simulink model "sim2"  (R2021a)
settings: Solver=ode4  StartTime=0.0  StopTime=2  RelTol=1e-3
libraries: spsVoltageMeasurementLib x7, spsIGBTDiodeLib x6, spsSeriesRLCBranchLib x5, spsCurrentMeasurementLib x4, spsACVoltageSourceLib x3, spsabctodq0Lib x2, spsGroundLib x2, simulink x1, spsdq0toabcLib x1, spspowerguiLib x1
settings Model: Creator=aks  LastModifiedBy=aks
settings SolverCC: ZeroCrossControl=DisableAll
settings DataIOCC: Refine=100

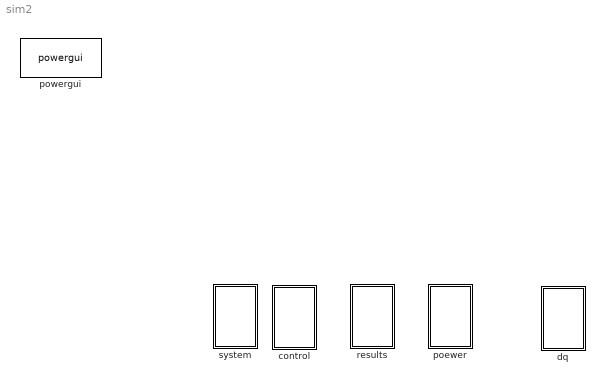
== system sim2 ==
  control : Subsystem
  dq : Subsystem
  poewer : Subsystem
  powergui : spspowerguiLib/powergui  Priority=1  SimulationMode=Discrete  SampleTime=1e-6  frequency=60  Iterations=50  frequencyindice=50  Pbase=100e6  ErrMax=1e-4  UnitsV=kV  UnitsW=MW  buscounter=0  FunctionMessages=off  echomessages=off  EnableUseOfTLC=off  CurrentSourceSwitches=off  DisableSnubberDevices=off  DisableRonSwitches=off  DisableVfSwitches=off  DisplayEquations=off  AutomaticDiscreteSolvers=off  SolverType=Tustin/Backward Euler (TBE)  Interpol=off  ExternalGateDelay=off  methode=off  Ts=100  x0status=blocks  SPID=on  SwTol=0  HookPort=off  NonlinearTolerance=1e-4  nMaxIteration=100  ContinueOnMaxIteration=off  RestoreLinks=warning  ResistiveCurrentMeasurement=off  Frange=[0:2:500]  Ylog=off  Xlog=on  ShowGrid=off  save=off  variable=ZData  structure=0  ZoomFFT=off  StartTime=0.0  cycles=1  DisplayStyle=1  fundamental=60  FreqAxis=off  MaxFrequency=1000  frequencyindicesteady=1  RmsSteady=1  display=off
  results : Subsystem
  system : Subsystem

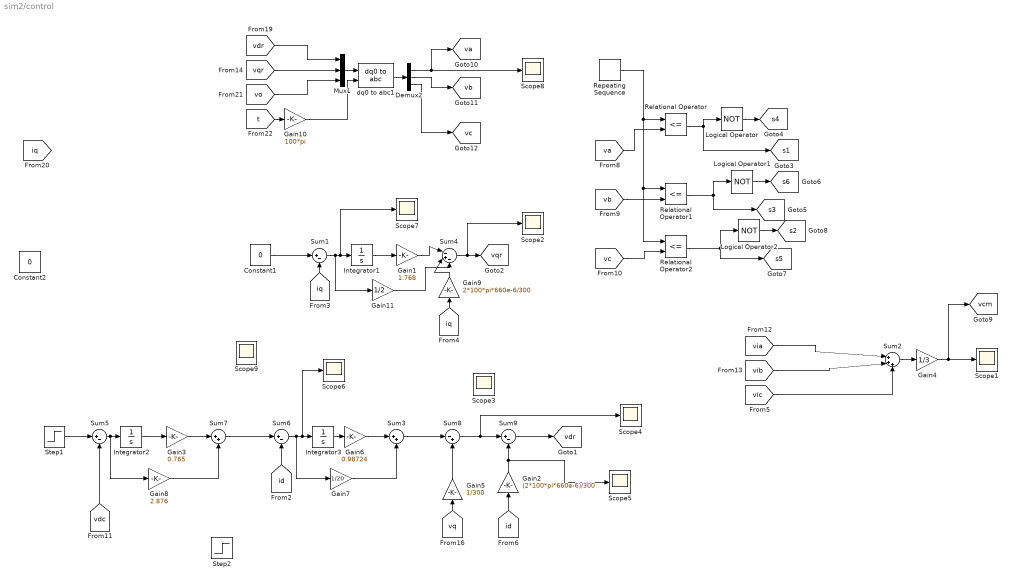
== system sim2/control ==
  Constant1 : Constant  Value=0
  Constant2 : Constant  Value=0
  Demux2 : Demux  Outputs=3
  Gain1 : Gain  Gain=1.768
  Gain10 : Gain  Gain=100*pi
  Gain11 : Gain  Gain=1/2
  Gain2 : Gain  Gain=(2*100*pi*660e-6)/300
  Gain3 : Gain  Gain=0.765
  Gain4 : Gain  Gain=1/3
  Gain5 : Gain  Gain=1/300
  Gain6 : Gain  Gain=0.98724
  Gain7 : Gain  Gain=1/20
  Gain8 : Gain  Gain=2.876
  Gain9 : Gain  Gain=2*100*pi*660e-6/300
  Integrator1 : Integrator
  Integrator2 : Integrator
  Integrator3 : Integrator
  Logical Operator : Logic  Operator=NOT  AllPortsSameDT=off  OutDataTypeStr=boolean
  Logical Operator1 : Logic  Operator=NOT  AllPortsSameDT=off  OutDataTypeStr=boolean
  Logical Operator2 : Logic  Operator=NOT  AllPortsSameDT=off  OutDataTypeStr=boolean
  Mux1 : Mux  Inputs=3
  Relational Operator : RelationalOperator  Operator=<=  OutDataTypeStr=boolean  RndMeth=Simplest
  Relational Operator1 : RelationalOperator  Operator=<=  OutDataTypeStr=boolean  RndMeth=Simplest
  Relational Operator2 : RelationalOperator  Operator=<=  OutDataTypeStr=boolean  RndMeth=Simplest
  Repeating Sequence : simulink/Sources/Repeating Sequence  rep_seq_t=[0 (1/20000) (1/10000) (3/20000) (1/5000)]  rep_seq_y=[0 1 0 -1 0]
  Scope{1..9} (9 alike) : Scope
  Step1 : Step  Before=800  After=400  SampleTime=0
  Step2 : Step  Before=0.4  After=0.6  SampleTime=0
  Sum{1,5..6,9} (4 alike) : Sum  Inputs=|+-
  Sum2 : Sum  Inputs=|+++
  Sum3 : Sum  Inputs=|++
  Sum4 : Sum  Inputs=|-+-
  Sum7 : Sum  Inputs=|++
  Sum8 : Sum  Inputs=|-+
  dq0 to abc1 : spsdq0toabcLib/dq0 to abc  Alignment=90 degrees behind phase A axis
  tag scope: s1=global, s2=global, s3=global, s4=global, s5=global, s6=global, va=global, vb=global, vc=global, vcm=global, vdr=global, vqr=global
  wires:
  Sum1/1 -> Gain11/1, Scope7/1, Integrator1/1
  Integrator1/1 -> Gain1/1
  Gain1/1 -> Sum4/1
  Constant1/1 -> Sum1/1
  Repeating Sequence/1 -> Relational Operator2/1, Relational Operator1/1, Relational Operator/1
  Relational Operator/1 -> [s1], Logical Operator/1
  Logical Operator/1 -> [s4]
  Logical Operator1/1 -> [s6]
  Relational Operator1/1 -> Logical Operator1/1, [s3]
  Relational Operator2/1 -> Logical Operator2/1, [s5]
  Logical Operator2/1 -> [s2]
  Step1/1 -> Sum5/1
  [vdc] -> Sum5/2
  [id] -> Gain2/1
  [iq] -> Gain9/1
  Gain9/1 -> Sum4/2
  Sum6/1 -> Gain7/1, Scope6/1, Integrator3/1
  Integrator3/1 -> Gain6/1
  Sum8/1 -> Scope4/1, Sum9/1
  Gain2/1 -> Scope5/1, Sum9/2
  Gain5/1 -> Sum8/2
  Sum5/1 -> Gain8/1, Integrator2/1
  Integrator2/1 -> Gain3/1
  [vic] -> Sum2/3
  [vib] -> Sum2/2
  [via] -> Sum2/1
  Sum2/1 -> Gain4/1
  Gain4/1 -> [vcm], Scope1/1
  [t] -> Gain10/1
  dq0 to abc1/1 -> Demux2/1
  Gain10/1 -> dq0 to abc1/2
  [vo] -> Mux1/3
  Mux1/1 -> dq0 to abc1/1
  Demux2/1 -> Scope8/1, [va]
  Demux2/2 -> [vb]
  Demux2/3 -> [vc]
  [va] -> Relational Operator/2
  [vb] -> Relational Operator1/2
  [vc] -> Relational Operator2/2
  [vq] -> Gain5/1
  [vdr] -> Mux1/1
  [vqr] -> Mux1/2
  Sum9/1 -> [vdr]
  Sum4/1 -> Scope2/1, [vqr]
  Gain7/1 -> Sum3/2
  Gain6/1 -> Sum3/1
  Sum3/1 -> Sum8/1
  [iq] -> Sum1/2
  [id] -> Sum6/2
  Gain3/1 -> Sum7/1
  Gain8/1 -> Sum7/2
  Sum7/1 -> Sum6/1
  Gain11/1 -> Sum4/3

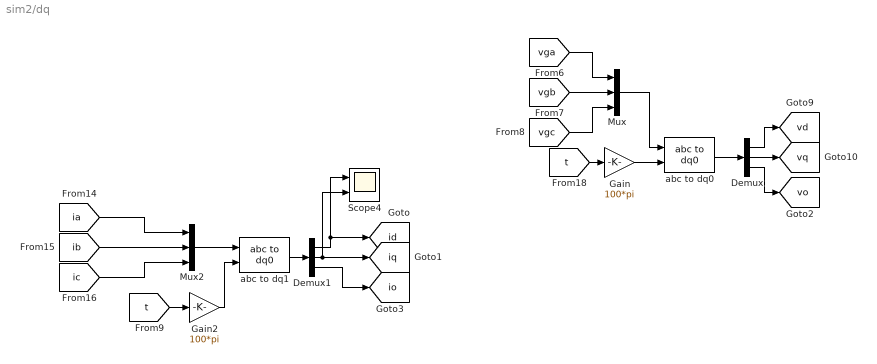
== system sim2/dq ==
  Demux : Demux  Outputs=3
  Demux1 : Demux  Outputs=3
  Gain : Gain  Gain=100*pi
  Gain2 : Gain  Gain=100*pi
  Mux : Mux  Inputs=3
  Mux2 : Mux  Inputs=3
  Scope4 : Scope  NumInputPorts=2
  abc to dq0 : spsabctodq0Lib/abc to dq0  Alignment=90 degrees behind phase A axis
  abc to dq1 : spsabctodq0Lib/abc to dq0  Alignment=90 degrees behind phase A axis
  tag scope: id=global, io=global, iq=global, vd=global, vo=global, vq=global
  wires:
  [t] -> Gain/1
  Demux/2 -> [vq]
  Demux/1 -> [vd]
  [vgb] -> Mux/2
  Gain/1 -> abc to dq0/2
  [vga] -> Mux/1
  [vgc] -> Mux/3
  Mux/1 -> abc to dq0/1
  abc to dq0/1 -> Demux/1
  Demux/3 -> [vo]
  Mux2/1 -> abc to dq1/1
  [ia] -> Mux2/1
  [ic] -> Mux2/3
  [ib] -> Mux2/2
  [t] -> Gain2/1
  Gain2/1 -> abc to dq1/2
  abc to dq1/1 -> Demux1/1
  Demux1/1 -> Scope4/1, [id]
  Demux1/2 -> [iq], Scope4/2
  Demux1/3 -> [io]

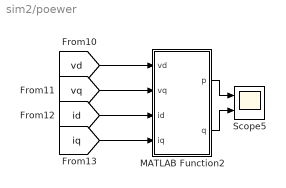
== system sim2/poewer ==
  MATLAB Function2 : MATLAB Function  TreatAsAtomicUnit=on
  Scope5 : Scope  NumInputPorts=2
  wires:
  MATLAB Function2/2(q) -> Scope5/2
  [vq] -> MATLAB Function2/2(vq)
  [iq] -> MATLAB Function2/4(iq)
  [vd] -> MATLAB Function2/1(vd)
  MATLAB Function2/1(p) -> Scope5/1
  [id] -> MATLAB Function2/3(id)

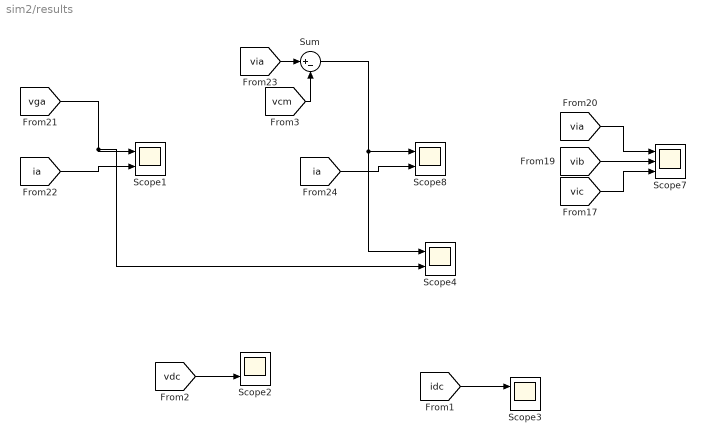
== system sim2/results ==
  Scope{1..4,8} (5 alike) : Scope  NumInputPorts=2
  Scope7 : Scope  NumInputPorts=3
  Sum : Sum  Inputs=|+-
  wires:
  [vga] -> Scope4/2, Scope1/1
  [ia] -> Scope8/2
  [vic] -> Scope7/3
  [ia] -> Scope1/2
  [vib] -> Scope7/2
  [via] -> Scope7/1
  [vdc] -> Scope2/2
  [idc] -> Scope3/1
  [via] -> Sum/1
  [vcm] -> Sum/2
  Sum/1 -> Scope4/1, Scope8/1

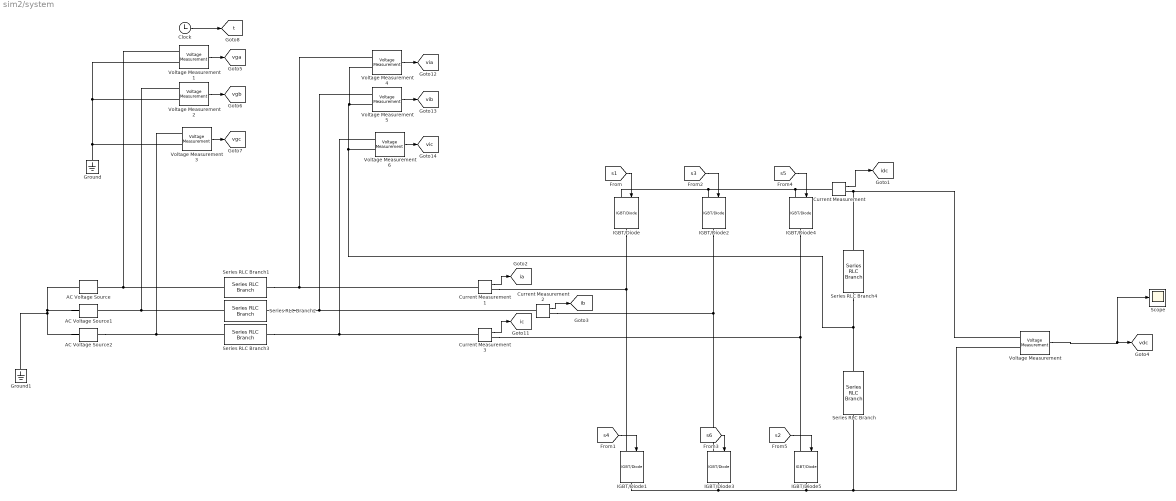
== system sim2/system ==
  AC Voltage Source : spsACVoltageSourceLib/AC Voltage Source  Amplitude=168*sqrt(2)  Phase=0  Frequency=50  SampleTime=0  Measurements=None  BusType=swing  Pref=10e3  Qref=0  Qmin=-inf  Qmax=+inf
  AC Voltage Source1 : spsACVoltageSourceLib/AC Voltage Source  Amplitude=168*sqrt(2)  Phase=-120  Frequency=50  SampleTime=0  Measurements=None  BusType=swing  Pref=10e3  Qref=0  Qmin=-inf  Qmax=+inf
  AC Voltage Source2 : spsACVoltageSourceLib/AC Voltage Source  Amplitude=168*sqrt(2)  Phase=120  Frequency=50  SampleTime=0  Measurements=None  BusType=swing  Pref=10e3  Qref=0  Qmin=-inf  Qmax=+inf
  Clock : Clock
  Current Measurement{,1..3} (4 alike) : spsCurrentMeasurementLib/Current Measurement  PhasorSimulation=off  OutputType=Complex  PSBequivalent=0
  Ground : spsGroundLib/Ground  LConnTagsString=a
  Ground1 : spsGroundLib/Ground  LConnTagsString=a
  IGBT/Diode{,1..5} (6 alike) : spsIGBTDiodeLib/IGBT//Diode  Ron=1e-3  Rs=1e5  Cs=inf  Measurements=off
  Scope : Scope
  Series RLC Branch : spsSeriesRLCBranchLib/Series RLC Branch  LConnTagsString=__new0  RConnTagsString=__new0  BranchType=C  Resistance=10000  Inductance=1e-3  SetiL0=off  InitialCurrent=0  Capacitance=2*(6750e-6)  Setx0=on  InitialVoltage=0  Measurements=None
  Series RLC Branch1 : spsSeriesRLCBranchLib/Series RLC Branch  LConnTagsString=__new0  RConnTagsString=__new0  BranchType=RL  Resistance=2e-3  Inductance=660e-6  SetiL0=off  InitialCurrent=0  Capacitance=1e-6  Setx0=off  InitialVoltage=0  Measurements=None
  Series RLC Branch2 : spsSeriesRLCBranchLib/Series RLC Branch  LConnTagsString=__new0  RConnTagsString=__new0  BranchType=RL  Resistance=2e-3  Inductance=660e-6  SetiL0=off  InitialCurrent=0  Capacitance=1e-6  Setx0=off  InitialVoltage=0  Measurements=None
  Series RLC Branch3 : spsSeriesRLCBranchLib/Series RLC Branch  LConnTagsString=__new0  RConnTagsString=__new0  BranchType=RL  Resistance=2e-3  Inductance=660e-6  SetiL0=off  InitialCurrent=0  Capacitance=1e-6  Setx0=off  InitialVoltage=0  Measurements=None
  Series RLC Branch4 : spsSeriesRLCBranchLib/Series RLC Branch  LConnTagsString=__new0  RConnTagsString=__new0  BranchType=C  Resistance=10000  Inductance=1e-3  SetiL0=off  InitialCurrent=0  Capacitance=2*(6750e-6)  Setx0=on  InitialVoltage=0  Measurements=None
  Voltage Measurement{,1..6} (7 alike) : spsVoltageMeasurementLib/Voltage Measurement  PhasorSimulation=off  OutputType=Complex  PSBequivalent=0
  tag scope: ia=global, ib=global, ic=global, idc=global, t=global, vdc=global, vga=global, vgb=global, vgc=global, via=global, vib=global, vic=global
  wires:
  Current Measurement2/1 -> [ib]
  Voltage Measurement2/1 -> [vgb]
  Voltage Measurement3/1 -> [vgc]
  Voltage Measurement/1 -> [vdc], Scope/1
  Clock/1 -> [t]
  Voltage Measurement5/1 -> [vib]
  Current Measurement3/1 -> [ic]
  Voltage Measurement4/1 -> [via]
  Voltage Measurement6/1 -> [vic]
  Current Measurement/1 -> [idc]
  Current Measurement1/1 -> [ia]
  Voltage Measurement1/1 -> [vga]
  [s1] -> IGBT/Diode/1
  [s3] -> IGBT/Diode2/1
  [s5] -> IGBT/Diode4/1
  [s2] -> IGBT/Diode5/1
  [s6] -> IGBT/Diode3/1
  [s4] -> IGBT/Diode1/1
  connections:
  IGBT/Diode/RConn1 -- Current Measurement1/RConn1 -- IGBT/Diode1/LConn1
  Current Measurement/RConn1 -- Voltage Measurement/LConn1 -- Series RLC Branch4/LConn1
  IGBT/Diode/LConn1 -- Current Measurement/LConn1 -- IGBT/Diode4/LConn1 -- IGBT/Diode2/LConn1
  Series RLC Branch2/RConn1 -- Voltage Measurement5/LConn1 -- Current Measurement2/LConn1
  Series RLC Branch3/RConn1 -- Voltage Measurement6/LConn1 -- Current Measurement3/LConn1
  IGBT/Diode1/RConn1 -- IGBT/Diode3/RConn1 -- Voltage Measurement/LConn2 -- Series RLC Branch/RConn1 -- IGBT/Diode5/RConn1
  Series RLC Branch1/RConn1 -- Voltage Measurement4/LConn1 -- Current Measurement1/LConn1
  IGBT/Diode4/RConn1 -- IGBT/Diode5/LConn1 -- Current Measurement3/RConn1
  Ground1/LConn1 -- AC Voltage Source2/LConn1 -- AC Voltage Source/LConn1 -- AC Voltage Source1/LConn1
  Series RLC Branch1/LConn1 -- Voltage Measurement1/LConn1 -- AC Voltage Source/RConn1
  Series RLC Branch2/LConn1 -- Voltage Measurement2/LConn1 -- AC Voltage Source1/RConn1
  IGBT/Diode2/RConn1 -- Current Measurement2/RConn1 -- IGBT/Diode3/LConn1
  Ground/LConn1 -- Voltage Measurement1/LConn2 -- Voltage Measurement2/LConn2 -- Voltage Measurement3/LConn2
  AC Voltage Source2/RConn1 -- Series RLC Branch3/LConn1 -- Voltage Measurement3/LConn1
  Voltage Measurement4/LConn2 -- Series RLC Branch/LConn1 -- Series RLC Branch4/RConn1 -- Voltage Measurement6/LConn2 -- Voltage Measurement5/LConn2

== matlab function sim2/poewer/MATLAB Function2 ==
  data: vd input; p output; vq input; id input; iq input; q output
function [p,q]= fcn(vd,vq,id,iq)
p= (vd*id+vq*iq);
q=(vq*id-vd*iq);
